simulink model "plant_test"  (R2025b)
settings: Solver=ode45  StartTime=0.0  StopTime=10.0  RelTol=1e-3
InitFcn:
  | p = params()
undefined symbols (not defined in the file or in its folder): x0_omega, x0_q, x0_r, x0_v
settings Model: Creator=C4gie  LastModifiedBy=C4gie

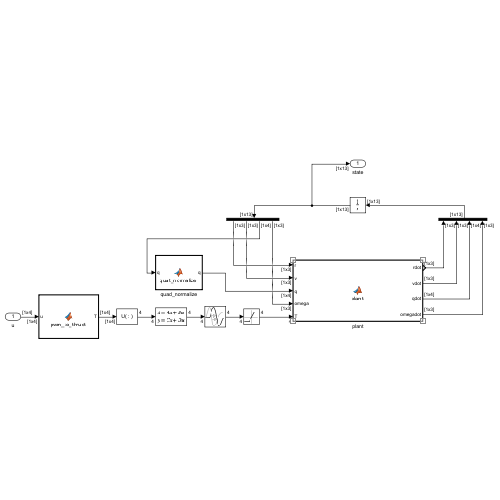
[thumbnail: Simulink's stored preview of the top-level diagram]
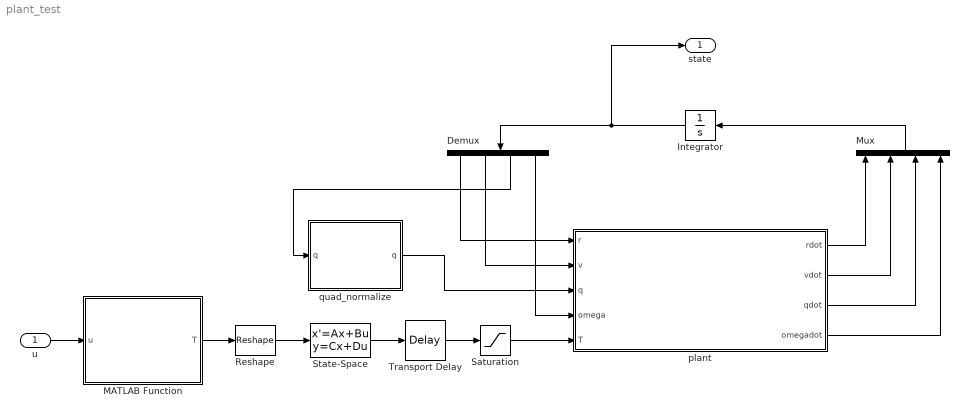
== system plant_test ==
  u : Inport  PortDimensions=[1 4]
  Demux : Demux
  Integrator : Integrator  InitialCondition=[x0_r, x0_v, x0_q, x0_omega]
  MATLAB Function : MATLAB Function  TreatAsAtomicUnit=on
  Mux : Mux
  Reshape : Reshape
  Saturation : Saturate  UpperLimit=p.motor.max_thrust  LowerLimit=p.motor.min_thrust
  State-Space : StateSpace  A=-1/p.motor.tau * eye(4)  B=p.motor.k/p.motor.tau * eye(4)  C=eye(4)  D=zeros(4)  InitialCondition=0
  Transport Delay : TransportDelay  DelayTime=p.motor.delay
  plant : MATLAB Function  TreatAsAtomicUnit=on
  quad_normalize : MATLAB Function  TreatAsAtomicUnit=on
  state : Outport
  wires:
  u/1 -> MATLAB Function/1(u)
  plant/1(rdot) -> Mux/1
  plant/2(vdot) -> Mux/2
  plant/3(qdot) -> Mux/3
  plant/4(omegadot) -> Mux/4
  Mux/1 -> Integrator/1
  Integrator/1 -> Demux/1, state/1
  Demux/1 -> plant/1(r)
  Demux/2 -> plant/2(v)
  Demux/3 -> quad_normalize/1("q ")
  Demux/4 -> plant/4(omega)
  Reshape/1 -> State-Space/1
  Transport Delay/1 -> Saturation/1
  Saturation/1 -> plant/5(T)
  State-Space/1 -> Transport Delay/1
  MATLAB Function/1(T) -> Reshape/1
  quad_normalize/1(q) -> plant/3(q)

== matlab function plant_test/MATLAB Function ==
  data: u input; T output; p parameter
function T = pwm_to_thrust(u, p)
    T = pwm_to_thrust(u, p);
end

== matlab function plant_test/plant ==
  data: r input size=[1 3]; rdot output size=[1 3]; v input size=[1 3]; q input size=[1 4]; omega input size=[1 3]; T input size=[1 4]; vdot output size=[1 3]; qdot output size=[1 4]; omegadot output size=[1 3]; p parameter
function [rdot, vdot, qdot, omegadot] = plant(r, v, q, omega, T, p)
    [rdot, vdot, qdot, omegadot] = plant(r, v, q, omega, T, p);
end

== matlab function plant_test/quad_normalize ==
  data: q input; q output
function q = quat_normalize(q)
    q = quat_normalize(q);
end
